simulink model "Soundtest"  (R2021a)
settings: Solver=FixedStepAuto  StartTime=0.0  StopTime=90  RelTol=1e-3
undefined symbols (not defined in the file): fdesignblkfcn, gcbh
libraries: simulink x25, simulink_extras x14, hdlsllib x9, eeGeneralControl x5, dspvision x4, commrandsrc3 x4, commutil2 x1
(part 2 of 5)

== system Soundtest/Detection_Block/Ambulance_Detectors/Ambulance_Detector_1/Bandpass_Filter ==
  In : Inport
  Generated Filter Block : DiscreteFir  Tag=BlockMethodSubSystem  Coefficients=[-2.79694201365472481e-06 -3.87049446814999036e-06 -5.00158247766914371e-06 -6.14380105789789502e-06 -7.2459808304134087e-06 -8.25406234390509597e-06 -9.11319308586671339e-06 -9.76997093709944376e-06 -1.01747487281602967e-05 -1.02839086178427031e-05 -1.00620125785226668e-05 -9.48373655919813677e-06 -8.53550097688946083e-06 -7.21671898103937179e-06 -5.54059621051784922e-06 -3.53443113698389131e-06 -1.2393830425519445e-06 1.29030542563434238e-06 3.98862308366914354e-06 6.77961288947415371e-06 9.57965190097747724e-06 1.23001182146055349e-05 1.48503569944929628e-05 1.71408430176351764e-05 1.90864260531815449e-05 2.06095384143192243e-05 2.16432415686200905e-05 2.21339909976899554e-05 2.20440056065158562e-05 2.13531397538254356e-05 2.00601720741799961e-05 1.81834451761402261e-05 1.57608133487020129e-05 1.28488807674219555e-05 9.52153942561907054e-06 5.8678431087062646e-06 1.98928012422263547e-06 -2.00346786024161938e-06 -5.99417164866355608e-06 -9.86497762467341039e-06 -1.35004670800181085e-05 -1.67917022012702403e-05 -1.9640106265071695e-05 -2.1961028573705717e-05 -2.36868535377790768e-05 -2.47695278732178369e-05 -2.51823996875163741e-05 -2.49212876290293358e-05 -2.40047264096255282e-05 -2.24733658635958074e-05 -2.03885331212903577e-05 -1.7830000212557345e-05 -1.48930311891250262e-05 -1.16848123913572854e-05 -8.3203955672950958e-06 -4.91830507331181662e-06 -1.59597639409599083e-06 1.53479704018670466e-06 4.37222881400083005e-06 6.82854044976360572e-06 8.83343364402858192e-06 1.03368870954248213e-05 1.13111553363794665e-05 1.17518764974663847e-05 1.16782297811805203e-05 1.11321203530282987e-05 1.01764079732926682e-05 8.89223449549756118e-06 7.37554280885767529e-06 5.73291438192426558e-06 4.07688283270793433e-06 2.52090560445581117e-06 1.17419375682102387e-06 1.36610221359657797e-07 -5.06150968459953747e-07 -6.86898255270498555e-07 -3.60597420163867627e-07 4.92821086374417478e-07 1.86664115202708117e-06 3.72662886517752458e-06 6.01145046748294341e-06 8.63425687774939188e-06 1.14854047331146403e-05 1.44362373773881303e-05 1.73438045710222901e-05 2.00563587136347906e-05 2.24194297665968217e-05 2.42822523759423277e-05 2.55042982241134053e-05 2.59616553890582986e-05 2.55529951278251259e-05 2.42048753230521464e-05 2.18761487354299259e-05 1.85612726965631428e-05 1.42923540705503802e-05 9.13980796399914515e-06 3.2115592076941484e-06 -3.34922976258696738e-06 -1.0367864365161805e-05 -1.76431599044067056e-05 -2.49536692301457939e-05 -3.2064895386809181e-05 -3.87372454408702022e-05 -4.47344468429953197e-05 -4.98321227302567029e-05 -5.38262086927083808e-05 -5.65408915027389991e-05 -5.78357604770919412e-05 -5.76118843868699923e-05 -5.58165605566082881e-05 -5.24465269488202506e-05 -4.75494811391230854e-05 -4.12238102960588154e-05 -3.36165014234594803e-05 -2.49192688014066701e-05 -1.53630032278810278e-05 -5.21071272022592266e-06 5.25081576405278518e-06 1.57203516823559954e-05 2.58922287964519131e-05 3.54666699469802116e-05 4.41600548949931708e-05 5.17147531204384625e-05 5.79081534718841085e-05 6.25605467385878723e-05 6.55415548919008892e-05 6.67748507114721679e-05 6.62409720698814598e-05 6.3978104154734184e-05 6.00807778530942061e-05 5.46965106286090909e-05 4.80204945349394251e-05 4.02885115186891657e-05 3.17683259152970406e-05 2.27498652485579506e-05 1.35345506072571872e-05 4.424174874328587e-06 -4.2902507179268481e-06 -1.23392549359768952e-05 -1.9484853129405003e-05 -2.55292917600800093e-05 -3.03222424708878219e-05 -3.37661533085378972e-05 -3.58195329191550438e-05 -3.64980214686799241e-05 -3.58731868272229565e-05 -3.40690730072627874e-05 -3.12566165729195926e-05 -2.76461322864427076e-05 -2.34781482384107106e-05 -1.90129399277952608e-05 -1.45191693507717121e-05 -1.02620766994049663e-05 -6.49169688466738251e-06 -3.43157953159957002e-06 -1.26847878420452513e-06 -1.43448360992319755e-07 -1.44728704177271062e-07 -1.3027483570698131e-06 -3.58748313256776848e-06 -6.90832702852892273e-06 -1.11165315115320323e-05 -1.60101683978283941e-05 ...(+39832 chars)]  InputProcessing=Columns as channels (frame based)
  Out : Outport  VectorParamsAs1DForOutWhenUnconnected=off
  wires:
  In/1 -> Generated Filter Block/1
  Generated Filter Block/1 -> Out/1
